simulink model "relational_operator"  (R2022a)
settings: Solver=VariableStepAuto  StartTime=0.0  StopTime=10.0  RelTol=1e-3
settings Model: Creator=Home computer  LastModifiedBy=Home computer

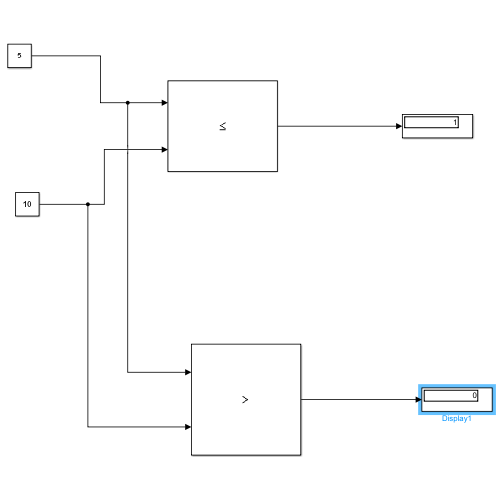
[thumbnail: Simulink's stored preview of the top-level diagram]
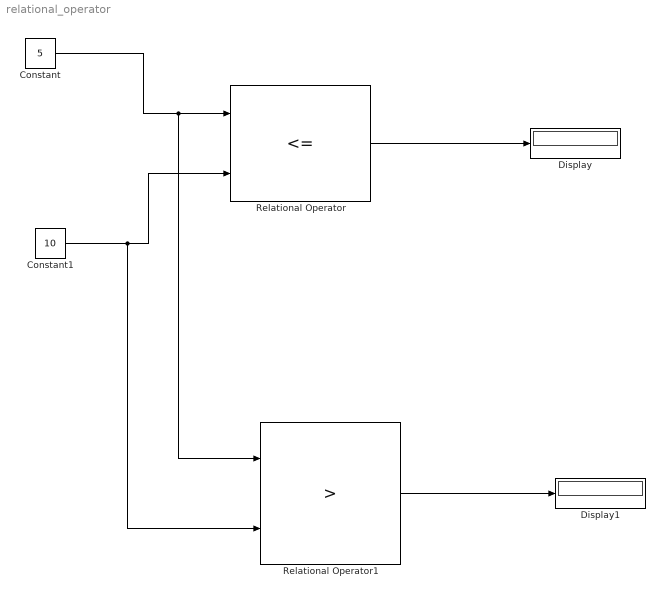
== system relational_operator ==
  Constant : Constant  Value=5
  Constant1 : Constant  Value=10
  Display : Display
  Display1 : Display
  Relational Operator : RelationalOperator  Operator=<=  OutDataTypeStr=boolean  RndMeth=Simplest  InputSameDT=off
  Relational Operator1 : RelationalOperator  Operator=>  OutDataTypeStr=boolean  RndMeth=Simplest  InputSameDT=off
  wires:
  Constant/1 -> Relational Operator1/1, Relational Operator/1
  Constant1/1 -> Relational Operator1/2, Relational Operator/2
  Relational Operator/1 -> Display/1
  Relational Operator1/1 -> Display1/1
